simulink library "lib_controls"  (Simulink 7.9)
settings: Solver=ode45  SolverMode=SingleTasking  StartTime=0.0  StopTime=10.0  RelTol=1e-3
undefined symbols (not defined in the file): amb_tmp, cs_charge_deplete_bool, cs_charge_pwr, cs_charge_trq, cs_clt_tmp, cs_decel_fc_off, cs_decel_regen_threshold, cs_dl_assist_trq_threshold, cs_dl_regen_trq_threshold, cs_electric_decel_spd, cs_electric_launch_spd, cs_electric_launch_spd_hi, cs_electric_launch_spd_lo, cs_eng_min_spd, cs_eng_on_soc, cs_fc_init_state, cs_fc_max_pwr_frac, cs_fc_min_pwr_frac, cs_fc_on, cs_fc_pwr_opt, cs_fc_spd_opt, cs_fuzzy_fuel_mode, cs_hi_soc, cs_hi_trq_frac, cs_lo_soc, cs_lo_trq_frac, cs_max_gc_spd, cs_max_pwr, cs_max_pwr_fall_rate, cs_max_pwr_rise_rate, cs_mc_assist_max_frac, cs_mc_assist_min_frac, cs_mc_assist_slope, cs_mc_regen_max_frac, cs_mc_regen_min_frac, cs_mc_regen_slope, cs_mean_eff, cs_mean_eff_bool, cs_min_gc_spd, cs_min_off_time, cs_min_pwr, cs_min_trq_frac, cs_mph_avg_time, cs_off_trq_frac, cs_plot_output, cs_pwr, cs_regen_avg_time, cs_scale_factor, cs_shutoff, cs_soc_range, cs_spd, cs_target_soc, cs_trq_to_soc_factor, cvt_locus_pwr, cvt_locus_spd, cyc_mph, enable_sim_stop_distance, enable_sim_stop_max_spd, enable_sim_stop_speed, enable_sim_stop_time ... (+110)
libraries: lib_controls x124, simulink3 x18, lib_etc x1
(part 3 of 17)

== system lib_controls/electric assist control strategy bal <cs> ==
  "trq and spd req'd into clutch (N*m, rad/s)" : Inport
  Constant : Constant  Value=0
  MinMax : MinMax  Function=max  Inputs=2  SaturateOnIntegerOverflow=on  InputSameDT=on
  Mux : Mux  Inputs=2
  SOC corrected  trq req'd (N*m) : Subsystem
  Selector : Selector  InputPortWidth=2  IndexOptions=Index vector (dialog)  Indices=2  OutputSizes=1
  Switch : Switch  Threshold=eps  SaturateOnIntegerOverflow=on  InputSameDT=on
  help : Subsystem
      settings: OpenFcn=web(['file:\\\' which('Parallel.htm')])
      mask Display: image(imread('doc_man.jpg'))
  minimum trq (N*m) : Subsystem
  "trq and spd req'd from engine (N*m, rad/s)" : Outport
  wires:
  SOC corrected  trq req'd (N*m)/1(SOC corrected  trq req'd (N*m)) -> MinMax/1
  MinMax/1 -> Switch/1
  "trq and spd req'd into clutch (N*m, rad/s)"/1 -> SOC corrected  trq req'd (N*m)/1("trq and spd req'd into trq coupler (N*m, rad/s)"), Selector/1, minimum trq (N*m)/1("trq and spd req'd into trq coupler (N*m, rad/s)")
  minimum trq (N*m)/1(minimum trq (N*m)) -> MinMax/2
  [engine_on] -> Switch/2
  Selector/1 -> Mux/2
  Mux/1 -> "trq and spd req'd from engine (N*m, rad/s)"/1
  Switch/1 -> Mux/1
  Constant/1 -> Switch/3

== system lib_controls/electric assist control strategy  CVT <cs> ==
  "trq and spd req'd into clutch (N*m, rad/s)" : Inport
  Block NOTES1 : Subsystem
      mask Display: disp('Block\nNOTES')
  Constant : Constant  Value=0
  Demux : Demux  Outputs=2
  Demux1 : Demux  Outputs=2
  FC trq and spd : Subsystem
  MinMax : MinMax  Function=max  Inputs=2  SaturateOnIntegerOverflow=on  InputSameDT=on
  Mux : Mux  Inputs=2
  Switch : Switch  Threshold=eps  SaturateOnIntegerOverflow=on  InputSameDT=on
  To Workspace : ToWorkspace  VariableName=cl_trq_in_r  SampleTime=-1
  To Workspace1 : ToWorkspace  VariableName=cl_spd_in_r  SampleTime=-1
  To Workspace2 : ToWorkspace  VariableName=cs_trq_in_r  SampleTime=-1
  To Workspace3 : ToWorkspace  VariableName=cs_spd_in_r  SampleTime=-1
  help : Subsystem
      settings: OpenFcn=web(['file:\\\' which('Parallel.htm')])
      mask Display: image(imread('doc_man.jpg'))
  minimum trq (Nm) : Subsystem
  mod pwr req : Subsystem
  raw pwr req : Product  Inputs=1  SaturateOnIntegerOverflow=on  RndMeth=Zero  InputSameDT=on  OutDataTypeStr=Inherit: Same as first input
  "trq and spd req'd from engine (N*m, rad/s)" : Outport
  wires:
  Demux1/2 -> Mux/2, To Workspace1/1
  Demux/2 -> To Workspace3/1
  FC trq and spd/1("engine torque and speed (Nm), (rad/s)") -> Demux/1
  mod pwr req/1(Out1) -> FC trq and spd/1(power req'd by FC (W))
  Demux1/1 -> To Workspace/1
  "trq and spd req'd into clutch (N*m, rad/s)"/1 -> Demux1/1, minimum trq (Nm)/1("trq and spd req'd into trq coupler (N*m, rad/s)"), raw pwr req/1
  Switch/1 -> To Workspace2/1, Mux/1
  minimum trq (Nm)/1(minimum trq (N*m)) -> MinMax/1
  Demux/1 -> MinMax/2
  Mux/1 -> "trq and spd req'd from engine (N*m, rad/s)"/1
  Constant/1 -> Switch/3
  MinMax/1 -> Switch/1
  [mode] -> FC trq and spd/3(Mode)
  [engine_on] -> FC trq and spd/2(FC on), Switch/2
  raw pwr req/1 -> mod pwr req/1(In1)

== system lib_controls/fuel cell adaptive <cs> ==
  power req'd by bus (W) : Inport
  Delta SOC expected from regen : Subsystem
  Demux : Demux  Outputs=2
  Logical Operator : Logic
  Memory : Memory
  Minimize energy : S-Function  FunctionName=sfun_fuelcell_adapt  Parameters=cs_max_pwr_rise_rate,cs_max_pwr_fall_rate,fc_fuel_lhv,cs_shutoff,cs_min_pwr,cs_max_pwr,cs_mean_eff_bool,cs_mean_eff,cs_plot_output  EnableBusSupport=off
  Mux : Mux  Inputs=8
  SOC regulation factor : Subsystem
  engine pwr (W) : Outport
  tag scope: engine_on=global
  wires:
  power req'd by bus (W)/1 -> Mux/1, Delta SOC expected from regen/1(Power req'd by bus (W))
  Mux/1 -> Minimize energy/1
  [SOC] -> Mux/3, SOC regulation factor/1(In1), Delta SOC expected from regen/2(Soc)
  Minimize energy/1 -> Demux/1
  [key_on] -> Logical Operator/2
  Demux/2 -> Logical Operator/1
  Demux/1 -> engine pwr (W)/1
  Logical Operator/1 -> [engine_on]
  SOC regulation factor/1(Out1) -> Mux/4
  [ess_max_pwr] -> Mux/5
  [ess_max_chg_pwr] -> Mux/6
  [ess_tmp] -> Mux/7
  Memory/1 -> Mux/8
  [fc_pwr_out_a] -> Memory/1
  Delta SOC expected from regen/1(Delta SOC regen) -> Mux/2

== system lib_controls/fuel cell control strategy <cs> ==
  power req'd by bus (W) : Inport
  FC on : Subsystem
  "FC pwr command, modified by SOC" : Subsystem
  "FC pwr command, w/ limits enforced" : Subsystem
  Product : Product  SaturateOnIntegerOverflow=on  RndMeth=Zero  InputSameDT=on  OutDataTypeStr=Inherit: Same as first input
  Relational Operator : RelationalOperator  InputSameDT=on
  pwr req'd from FC to supply pwr req'd at bus (W) : Subsystem
  engine pwr (W) : Outport  InitialOutput=0
  tag scope: engine_on=global
  wires:
  power req'd by bus (W)/1 -> FC on/4(bus pwr req), "FC pwr command, modified by SOC"/3(pwr req'd at bus (W)), Relational Operator/1, pwr req'd from FC to supply pwr req'd at bus (W)/1(power req'd by bus (W))
  [ess_max_pwr] -> Relational Operator/2
  Product/1 -> engine pwr (W)/1
  pwr req'd from FC to supply pwr req'd at bus (W)/1(pwr req'd of FC (W)) -> "FC pwr command, modified by SOC"/2(raw pwr command (W))
  "FC pwr command, w/ limits enforced"/1(limited FC pwr command (W)) -> Product/2
  Relational Operator/1 -> FC on/1(ess max pwr would be insufficient), "FC pwr command, w/ limits enforced"/1(ess max pwr would be insufficient)
  [SOC] -> "FC pwr command, modified by SOC"/1(SOC), FC on/2(SOC), "FC pwr command, w/ limits enforced"/2(SOC)
  "FC pwr command, modified by SOC"/1(pwr command modifed for SOC (W)) -> "FC pwr command, w/ limits enforced"/3(FC pwr command), FC on/3(FC pwr command)
  FC on/1(FC on) -> [engine_on], Product/1

== system lib_controls/fuel cell <cs> config ==
  power req'd by bus (W) : Inport
  fuel cell adaptive <cs> : lib_controls/fuel cell adaptive <cs>
  engine pwr (W) : Outport
  wires:
  power req'd by bus (W)/1 -> fuel cell adaptive <cs>/1
  fuel cell adaptive <cs>/1 -> engine pwr (W)/1

== system lib_controls/par <cs> config ==
  "trq and spd req'd into clutch (N*m, rad/s)" : Inport
  electric assist control strategy <cs> : lib_controls/electric assist control strategy <cs>
  "trq and spd req'd from engine (N*m, rad/s)" : Outport
  wires:
  "trq and spd req'd into clutch (N*m, rad/s)"/1 -> electric assist control strategy <cs>/1
  electric assist control strategy <cs>/1 -> "trq and spd req'd from engine (N*m, rad/s)"/1

== system lib_controls/par <vc> config ==
  <vc> par : lib_controls/<vc> par
  clutch state : Outport
  wires:
  <vc> par/1 -> clutch state/1

== system lib_controls/series hybrid control stategy  <cs> ==
  power req'd by bus (W) : Inport
  FC on : Subsystem
  "FC pwr command, modified by SOC" : Subsystem
  "FC pwr command, w/ limits enforced" : Subsystem
  FC trq and spd : Subsystem
  Relational Operator : RelationalOperator  InputSameDT=on
  Selector : Selector  InputPortWidth=2  IndexOptions=Index vector (dialog)  Indices=2  OutputSizes=1
  power follower : Subsystem
      settings: OpenFcn=web(['file:\\\' which('Series.htm')]);
      mask Display: image(imread('doc_man.jpg'))
  pwr req'd from FC to supply pwr req'd at bus (W) : Subsystem
  thermostat : Subsystem
      settings: OpenFcn=web(['file:\\\' which('Series-therm.htm')]);
      mask Display: image(imread('doc_man.jpg'))
  "engine torque and speed (Nm), (rad/s)" : Outport  InitialOutput=0
  tag scope: engine_on=global, spd_command=global
  wires:
  Selector/1 -> [spd_command]
  FC trq and spd/1("engine torque and speed (Nm), (rad/s)") -> Selector/1, "engine torque and speed (Nm), (rad/s)"/1
  "FC pwr command, w/ limits enforced"/1(limited FC pwr command (W)) -> FC trq and spd/2(power req'd by FC (W))
  FC on/1(FC on) -> [engine_on], FC trq and spd/1(FC on)
  power req'd by bus (W)/1 -> FC on/4(bus pwr req), "FC pwr command, modified by SOC"/3(pwr req'd at bus (W)), Relational Operator/1, pwr req'd from FC to supply pwr req'd at bus (W)/1(power req'd by bus (W))
  [ess_max_pwr] -> Relational Operator/2
  Relational Operator/1 -> FC on/1(ess max pwr would be insufficient), "FC pwr command, w/ limits enforced"/1(ess max pwr would be insufficient)
  pwr req'd from FC to supply pwr req'd at bus (W)/1(pwr req'd of FC (W)) -> "FC pwr command, modified by SOC"/2(raw pwr command (W))
  "FC pwr command, modified by SOC"/1(pwr command modifed for SOC (W)) -> "FC pwr command, w/ limits enforced"/3(FC pwr command), FC on/3(FC pwr command)
  [SOC] -> FC on/2(SOC), "FC pwr command, w/ limits enforced"/2(SOC), "FC pwr command, modified by SOC"/1(SOC)

== system lib_controls/user contributed engine on (balanced parallel hybrid) ==
  trq req'd out of clutch (N*m) : Inport
  spd req'd out of clutch (N*m)1 : Inport  Port=2
  fc_spd_out_r : Inport  Port=3
  v_ave_req : Inport  Port=4
  clutch state : Inport  Port=5
  (--)2 : Constant  Value=fc_on
  (--)3 : Constant
  (--)4 : Constant  Value=cs_lo_soc
  Block NOTES : Subsystem
      mask Display: disp('Block\nNOTES')
  Constant1 : Constant  Value=vc_eng_warmup_time
  Constant2 : Constant  Value=engine_shutdown_delay
  Constant3 : Constant  Value=vc_launch_spd
  Constant4 : Constant
  Constant{5..7,9} (4 alike) : Constant  Value=0
  Constant8 : Constant
  Hit  Crossing1 : HitCross  HitCrossingDirection=rising
  Logical Operator10 : Logic  Inputs=3
  Logical Operator12 : Logic  Inputs=3
  Logical Operator2 : Logic
  Rate Limiter1 : RateLimiter  RisingSlewLimit=inf  FallingSlewLimit=-1/1
  Relational Operator1 : RelationalOperator  Operator=>  InputSameDT=on
  Saturation : Saturate  UpperLimit=max(fc_map_spd)*fc_spd_scale  LowerLimit=vc_idle_spd*vc_idle_bool
  Switch{,1..4} (5 alike) : Switch  Threshold=eps  SaturateOnIntegerOverflow=on  InputSameDT=on
  Terminator : Terminator
  Terminator1 : Terminator
  clutch disengaged : RelationalOperator  Operator===  InputSameDT=on
  clutch disengaged1 : RelationalOperator  Operator===  InputSameDT=on
  key_on : lib_controls/<vc> ISG bal shift by time CD3xx/engine on (balanced parallel hybrid)/key_on  MaskParam1=vc_key_on(:,1)  MaskParam2=vc_key_on(:,2)
  moving next time : RelationalOperator  Operator=>  InputSameDT=on
  moving next time1 : RelationalOperator  InputSameDT=on
  not moving : RelationalOperator  Operator===  InputSameDT=on
  repeated cycle time : lib_controls/<vc> ISG bal shift by time CD3xx/engine on (balanced parallel hybrid)/repeated cycle time  t=cyc_mph(:,1)  y=cyc_mph(:,1)
  repeated cycle:  speed required at end of NEXT step : lib_controls/<vc> ISG bal shift by time CD3xx/engine on (balanced parallel hybrid)/repeated cycle:  speed required at end of NEXT step  t=cyc_mph(:,1)  y=cyc_mph(:,2)
  engine on : Outport
  spd command  (rad/s) : Outport  Port=2
  key on : Outport  Port=3
  wires:
  trq req'd out of clutch (N*m)/1 -> Terminator/1
  spd req'd out of clutch (N*m)1/1 -> Terminator1/1
  Logical Operator2/1 -> Switch3/2
  Relational Operator1/1 -> Logical Operator2/2
  Switch3/1 -> Logical Operator12/3
  moving next time1/1 -> Logical Operator2/1
  (--)3/1 -> Switch3/3
  Constant1/1 -> Relational Operator1/2
  repeated cycle time/1 -> Relational Operator1/1
  [SOC] -> moving next time1/1
  key_on/1 -> Logical Operator12/2, key on/1  "ignition key is on"
  (--)2/1 -> Logical Operator12/1
  Constant3/1 -> Switch/1
  Switch/1 -> Saturation/1
  Logical Operator10/1 -> Switch/2
  fc_spd_out_r/1 -> Switch/3
  Saturation/1 -> Switch1/1
  clutch state/1 -> clutch disengaged/1
  Switch1/1 -> spd command  (rad/s)/1
  Constant7/1 -> Switch1/3
  Constant4/1 -> clutch disengaged/2
  v_ave_req/1 -> not moving/1
  Constant5/1 -> not moving/2
  repeated cycle:  speed required at end of NEXT step/1 -> moving next time/1, Switch2/2, clutch disengaged1/1
  Constant6/1 -> moving next time/2
  clutch disengaged/1 -> Logical Operator10/1
  not moving/1 -> Logical Operator10/2
  moving next time/1 -> Logical Operator10/3, Switch4/2
  (--)4/1 -> moving next time1/2
  Logical Operator12/1 -> Switch4/3
  Constant8/1 -> Switch4/1
  Switch4/1 -> engine on/1, Switch1/2
  Switch2/1 -> Switch3/1
  Constant2/1 -> Switch2/1
  Constant9/1 -> clutch disengaged1/2
  clutch disengaged1/1 -> Hit  Crossing1/1
  Hit  Crossing1/1 -> Rate Limiter1/1
  Rate Limiter1/1 -> Switch2/3

== system lib_controls/<vc> conv/clutch control ==
  shifting : Inport
  gb_trq_in_r : Inport  Port=2
  gb_spd_in_r : Inport  Port=3
  Block NOTES : Subsystem
      mask Display: disp('Block\nNOTES')
  Constant : Constant  Value=1e-3
  Constant1 : Constant  Value=vc_clutch_bool
  Constant2 : Constant  Value=vc_idle_spd
  Constant3 : Constant  Value=1e-3
  Constant4 : Constant  Value=vc_launch_spd
  Constant5 : Constant  Value=2.5
  Fcn: 1 if clutch disengaged 2 if clutch slipping 3 if clutch engaged : Fcn  Expr=u[1]+2*u[2]*(1-u[1])*(1-u[3])+3*u[3]*(1-u[1])
  Logical Operator : Logic
  Logical Operator1 : Logic  Operator=OR
  Memory : Memory  X0=1+(2*(cyc_mph(1,2)>0))
  Mux : Mux  Inputs=3
  Relational Operator : RelationalOperator  Operator=<=  InputSameDT=on
  Relational Operator1 : RelationalOperator  Operator=<  InputSameDT=on
  Relational Operator2 : RelationalOperator  Operator=>  InputSameDT=on
  Relational Operator3 : RelationalOperator  Operator=<  InputSameDT=on
  clutch disengaged : Logic  Operator=OR
  clutch engaged : Logic  Operator=NOR
  clutch slipping : Logic  Inputs=3
  clutch was NOT fully engaged during last time step : RelationalOperator  Operator=<  InputSameDT=on
  gearbox speed estimator : Subsystem
  clutch state : Outport
  wires:
  gearbox speed estimator/1(Out1) -> Relational Operator3/1, Relational Operator1/1
  gb_spd_in_r/1 -> gearbox speed estimator/1(gb_spd_in_r if no gear change)
  shifting/1 -> clutch disengaged/1
  Logical Operator/1 -> clutch disengaged/2
  gb_trq_in_r/1 -> Relational Operator2/1, Relational Operator/1
  Logical Operator1/1 -> Logical Operator/2
  Relational Operator/1 -> Logical Operator/1
  Constant/1 -> Relational Operator/2
  Constant1/1 -> Logical Operator1/1
  clutch was NOT fully engaged during last time step/1 -> clutch slipping/3
  Constant5/1 -> clutch was NOT fully engaged during last time step/2
  Memory/1 -> clutch was NOT fully engaged during last time step/1
  Relational Operator3/1 -> clutch slipping/2
  Constant4/1 -> Relational Operator3/2
  clutch slipping/1 -> Mux/2, clutch engaged/2
  Relational Operator2/1 -> clutch slipping/1
  Constant3/1 -> Relational Operator2/2
  Fcn: 1 if clutch disengaged 2 if clutch slipping 3 if clutch engaged/1 -> Memory/1, clutch state/1
  clutch disengaged/1 -> Mux/1, clutch engaged/1
  clutch engaged/1 -> Mux/3
  Mux/1 -> Fcn: 1 if clutch disengaged 2 if clutch slipping 3 if clutch engaged/1
  Constant2/1 -> Relational Operator1/2
  Relational Operator1/1 -> Logical Operator1/2

== system lib_controls/<vc> conv/config traction control ==
  time-average vehicle speed  req'd (m/s) : Inport
  vehicle speed at beginning of time  step (m/s) : Inport  Port=2
  total tractive force req'd (N) : Inport  Port=3
  traction control 2 axle : lib_controls/SubSystem/traction control 2 axle
  req'd force (N) : Outport
  req'd speed (m/s) : Outport  Port=2
  weight on front axle (N) : Outport  Port=3
  weight on rear axle (N) : Outport  Port=4
  front/total  traction ratio : Outport  Port=5
  wires:
  time-average vehicle speed  req'd (m/s)/1 -> traction control 2 axle/1
  vehicle speed at beginning of time  step (m/s)/1 -> traction control 2 axle/2
  total tractive force req'd (N)/1 -> traction control 2 axle/3
  traction control 2 axle/1 -> req'd force (N)/1
  traction control 2 axle/2 -> req'd speed (m/s)/1
  traction control 2 axle/3 -> weight on front axle (N)/1
  traction control 2 axle/4 -> weight on rear axle (N)/1
  traction control 2 axle/5 -> front/total  traction ratio/1

== system lib_controls/<vc> conv/engine control ==
  clutch state : Inport
  shifting : Inport  Port=2
  fc_spd_out_r : Inport  Port=3
  v_ave_req : Inport  Port=4
  Block NOTES : Subsystem
      mask Display: disp('Block\nNOTES')
  Constant : Constant  Value=1.1
  Constant1 : Constant  Value=vc_idle_bool
  Constant2 : Constant  Value=vc_launch_spd
  Constant3 : Constant
  Constant4 : Constant  Value=0
  Constant5 : Constant  Value=0
  Constant6 : Constant  Value=0
  Logical Operator1 : Logic
  Logical Operator2 : Logic  Operator=OR
  Logical Operator3 : Logic  Operator=OR
  Logical Operator7 : Logic
  Logical Operator8 : Logic  Inputs=3
  Memory : Memory
  Saturation : Saturate  UpperLimit=max(fc_map_spd)*fc_spd_scale  LowerLimit=vc_idle_spd*vc_idle_bool
  Switch : Switch  Threshold=eps  SaturateOnIntegerOverflow=on  InputSameDT=on
  Switch1 : Switch  Threshold=eps  SaturateOnIntegerOverflow=on  InputSameDT=on
  clutch disengaged : RelationalOperator  Operator===  InputSameDT=on
  clutch slipping or engaged : RelationalOperator  Operator=>  InputSameDT=on
  key_on : Subsystem  mask(Repeating table){t=vc_key_on(:,1), y=vc_key_on(:,2)}
      mask prompts: t "Time values:"; y "Output values:"
      mask help:
      | Repeating table.
      | Enter values of time and output for first cycle.
      mask init:
      | period = max(t);
      mask Help: Repeats cycle given in table. Time values should be monotonically increasing.
  moving next time : RelationalOperator  Operator=>  InputSameDT=on
  not moving : RelationalOperator  Operator===  InputSameDT=on
  repeated cycle:  speed required at end of NEXT step : Subsystem  mask(Forward looking repeating table){t=cyc_mph(:,1), y=cyc_mph(:,2)}
      mask prompts: t "Time values:"; y "Output values:"
      mask help:
      | Forward looking repeating table.
      | Enter values of time and output for first cycle.
      mask init:
      | period = max(t);
      mask Help: Repeats cycle given in table with a one time step forward offset. Time values should be monotonically increasing.
  engine on : Outport
  spd command  (rad/s) : Outport  Port=2
  key on : Outport  Port=3
  wires:
  key_on/1(out_1) -> key on/1, Logical Operator1/1
  Constant6/1 -> Switch1/3
  Switch1/1 -> spd command  (rad/s)/1
  Saturation/1 -> Switch1/1
  Logical Operator3/1 -> Switch1/2, Memory/1, engine on/1
  Switch/1 -> Saturation/1
  Constant2/1 -> Switch/1
  fc_spd_out_r/1 -> Switch/3
  Logical Operator8/1 -> Switch/2
  Constant4/1 -> not moving/2
  Constant3/1 -> clutch disengaged/2
  v_ave_req/1 -> not moving/1
  repeated cycle:  speed required at end of NEXT step/1(out_1) -> moving next time/1
  Constant5/1 -> moving next time/2
  Logical Operator7/1 -> Logical Operator3/2
  Memory/1 -> Logical Operator7/2
  shifting/1 -> Logical Operator7/1
  Logical Operator2/1 -> Logical Operator1/2
  Logical Operator1/1 -> Logical Operator3/1
  clutch slipping or engaged/1 -> Logical Operator2/1
  Constant/1 -> clutch slipping or engaged/2
  Constant1/1 -> Logical Operator2/2
  clutch state/1 -> clutch slipping or engaged/1, clutch disengaged/1
  moving next time/1 -> Logical Operator8/3
  not moving/1 -> Logical Operator8/2
  clutch disengaged/1 -> Logical Operator8/1

== system lib_controls/<vc> conv/gearbox  control ==
  note: default gear number
      | calculation
  note: default shifting
      | calculation
  note: default gear ratio
      | calculation
  note: gear ratio and shifting pre-muxed
  note: output changes depending
      | upon whether speed
      | dependent shifting is used
  note: local GOTO blocks:
  note: local GOTO blocks
  gb_trq_out_r : Inport
  gb_spd_out_r : Inport  Port=2
  prev. Pout/Pin : Inport  Port=3
  tires are at traction limit : Inport  Port=4
  Block NOTES : Subsystem
      mask Display: disp('Block\nNOTES')
  Constant : Constant
  Constant14 : Constant  Value=tx_speed_dep
  Constant15 : Constant  Value=tx_speed_dep
  Demux : Demux  Outputs=2
  Fcn : Fcn  Expr=1/u
  Fcn1 : Fcn  Expr=1/u
  Gain1 : Gain  Gain=-1  SaturateOnIntegerOverflow=on  OutDataTypeStr=Inherit: Same as input  ParamDataTypeStr=Inherit: Same as input
  Mux : Mux  Inputs=2
  Product2 : Product  Inputs=*/  SaturateOnIntegerOverflow=on  RndMeth=Zero  InputSameDT=on  OutDataTypeStr=Inherit: Same as first input
  Product3 : Product  SaturateOnIntegerOverflow=on  RndMeth=Zero  InputSameDT=on  OutDataTypeStr=Inherit: Same as first input
  Rate Limiter : RateLimiter  RisingSlewLimit=1/(gb_shift_delay+eps)  FallingSlewLimit=-1/(gb_shift_delay+eps)
  Saturation : Saturate  UpperLimit=1  LowerLimit=0.2
  Saturation1 : Saturate  UpperLimit=gb_gears_num  LowerLimit=1
  Speed Dependent Shifting : lib_controls/SubSystem/Speed Dependent Shifting
      settings: RTWFcnNameOpts=Auto  RTWFileNameOpts=Auto
  Switch : Switch  Threshold=eps  SaturateOnIntegerOverflow=on  InputSameDT=on
  Switch1 : Switch  Threshold=0.5  SaturateOnIntegerOverflow=on  InputSameDT=on
  Switch2 : Switch  Threshold=0.5  SaturateOnIntegerOverflow=on  InputSameDT=on
  allow downshift? : Subsystem
  current gear number : Sum  SaturateOnIntegerOverflow=on  InputSameDT=on  OutDataTypeStr=Inherit: Same as first input
  delta gear number : Switch  Threshold=eps  SaturateOnIntegerOverflow=on  InputSameDT=on
  downshift  command : Subsystem
  engine torque capability : Lookup  InputValues=fc_map_spd*fc_spd_scale  Table=fc_max_trq*fc_trq_scale+eps  SaturateOnIntegerOverflow=on
  est eng trq : Sum  SaturateOnIntegerOverflow=on  InputSameDT=on  OutDataTypeStr=Inherit: Same as first input
  gb_spd_in_r : Product  SaturateOnIntegerOverflow=on  RndMeth=Zero  InputSameDT=on  OutDataTypeStr=Inherit: Same as first input
  gear ratio : Lookup  InputValues=[1:length(gb_ratio)]  Table=gb_ratio  SaturateOnIntegerOverflow=on
  gear ratio1 : Lookup  InputValues=[1:length(gb_ratio)]  Table=gb_ratio  SaturateOnIntegerOverflow=on
  gearbox speed estimator : Subsystem
  load=T/ (maxT at spd) : Saturate  UpperLimit=1  LowerLimit=0
  prev gear number : Memory  X0=gb_num_init
  prev gear ratio : Memory  X0=gb_ratio(gb_num_init)
  shifting1 : Subsystem
  upshift  command : Subsystem
  ~gb_trq_in_r : Product  Inputs=3  SaturateOnIntegerOverflow=on  RndMeth=Zero  InputSameDT=on  OutDataTypeStr=Inherit: Same as first input
  "gear ratio, out" : Outport  InitialOutput=0
  "shifting, out" : Outport  Port=2  InitialOutput=0
  "gear number, out" : Outport  Port=3  InitialOutput=0
  wires:
  delta gear number/1 -> current gear number/2
  Switch/1 -> downshift  command/2(engine load), upshift  command/2(engine load)
  load=T/ (maxT at spd)/1 -> Switch/3
  est eng trq/1 -> Product2/1
  ~gb_trq_in_r/1 -> est eng trq/1
  gearbox speed estimator/1(Out1) -> upshift  command/3(engine speed), downshift  command/3(engine speed), engine torque capability/1
  allow downshift?/1(allow shift) -> Product3/1
  Product3/1 -> delta gear number/3
  Gain1/1 -> Product3/2
  prev gear ratio/1 -> Fcn1/1, gb_spd_in_r/2
  gear ratio/1 -> prev gear ratio/1
  gb_spd_in_r/1 -> gearbox speed estimator/1(gb_spd_in_r if no gear change)
  gb_spd_out_r/1 -> gb_spd_in_r/1
  Rate Limiter/1 -> gear ratio/1
  tires are at traction limit/1 -> Switch/2
  Constant/1 -> Switch/1
  Product2/1 -> load=T/ (maxT at spd)/1
  prev gear number/1 -> current gear number/1, downshift  command/1(prev gear number), upshift  command/1(prev gear number), allow downshift?/1(prev gearnum)
  Saturation1/1 -> shifting1/1(gear number), Rate Limiter/1, [def_gear_num], gear ratio1/1, prev gear number/1
  Fcn/1 -> ~gb_trq_in_r/2
  engine torque capability/1 -> Product2/2
  Fcn1/1 -> ~gb_trq_in_r/3
  downshift  command/1(command) -> Gain1/1
  upshift  command/1(command) -> delta gear number/2, delta gear number/1
  gb_trq_out_r/1 -> ~gb_trq_in_r/1
  prev. Pout/Pin/1 -> Saturation/1
  Saturation/1 -> Fcn/1
  current gear number/1 -> Saturation1/1
  gear ratio1/1 -> [def_gear_ratio]
  shifting1/1(out_1) -> [def_shifting]
  Constant15/1 -> Switch2/2
  [spd_dep_muxed] -> Switch2/1
  Mux/1 -> Switch2/3
  [def_gear_ratio] -> Mux/1
  [def_shifting] -> Mux/2
  [v_req_limited] -> Speed Dependent Shifting/1
  Speed Dependent Shifting/1 -> [spd_dep_muxed]
  Speed Dependent Shifting/2 -> [spd_dep_gear_num]
  Switch2/1 -> Demux/1
  Demux/1 -> "gear ratio, out"/1
  Demux/2 -> "shifting, out"/1
  Switch1/1 -> "gear number, out"/1
  Constant14/1 -> Switch1/2
  [spd_dep_gear_num] -> Switch1/1
  [def_gear_num] -> Switch1/3
  [acc_mech_trq_est] -> est eng trq/2

== system lib_controls/<vc> conv Saber custom/clutch control ==
  shifting : Inport
  gb_trq_in_r : Inport  Port=2
  gb_spd_in_r : Inport  Port=3
  Block NOTES : Subsystem
      mask Display: disp('Block\nNOTES')
  Constant : Constant  Value=1e-3
  Constant1 : Constant  Value=vc_clutch_bool
  Constant2 : Constant  Value=vc_idle_spd
  Constant3 : Constant  Value=1e-3
  Constant4 : Constant  Value=vc_launch_spd
  Constant5 : Constant  Value=2.5
  Fcn: 1 if clutch disengaged 2 if clutch slipping 3 if clutch engaged : Fcn  Expr=u[1]+2*u[2]*(1-u[1])*(1-u[3])+3*u[3]*(1-u[1])
  Logical Operator : Logic
  Logical Operator1 : Logic  Operator=OR
  Memory : Memory  X0=1+(2*(cyc_mph(1,2)>0))
  Mux : Mux  Inputs=3
  Relational Operator : RelationalOperator  Operator=<=  InputSameDT=on
  Relational Operator1 : RelationalOperator  Operator=<  InputSameDT=on
  Relational Operator2 : RelationalOperator  Operator=>  InputSameDT=on
  Relational Operator3 : RelationalOperator  Operator=<  InputSameDT=on
  clutch disengaged : Logic  Operator=OR
  clutch engaged : Logic  Operator=NOR
  clutch slipping : Logic  Inputs=3
  clutch was NOT fully engaged during last time step : RelationalOperator  Operator=<  InputSameDT=on
  gearbox speed estimator : Subsystem
  clutch state : Outport
  wires:
  Relational Operator1/1 -> Logical Operator1/2
  Constant2/1 -> Relational Operator1/2
  Mux/1 -> Fcn: 1 if clutch disengaged 2 if clutch slipping 3 if clutch engaged/1
  clutch engaged/1 -> Mux/3
  clutch disengaged/1 -> clutch engaged/1, Mux/1
  Fcn: 1 if clutch disengaged 2 if clutch slipping 3 if clutch engaged/1 -> clutch state/1, Memory/1
  Constant3/1 -> Relational Operator2/2
  Relational Operator2/1 -> clutch slipping/1
  clutch slipping/1 -> clutch engaged/2, Mux/2
  Constant4/1 -> Relational Operator3/2
  Relational Operator3/1 -> clutch slipping/2
  Memory/1 -> clutch was NOT fully engaged during last time step/1
  Constant5/1 -> clutch was NOT fully engaged during last time step/2
  clutch was NOT fully engaged during last time step/1 -> clutch slipping/3
  Constant1/1 -> Logical Operator1/1
  Constant/1 -> Relational Operator/2
  Relational Operator/1 -> Logical Operator/1
  Logical Operator1/1 -> Logical Operator/2
  gb_trq_in_r/1 -> Relational Operator/1, Relational Operator2/1
  Logical Operator/1 -> clutch disengaged/2
  shifting/1 -> clutch disengaged/1
  gb_spd_in_r/1 -> gearbox speed estimator/1(gb_spd_in_r if no gear change)
  gearbox speed estimator/1(Out1) -> Relational Operator1/1, Relational Operator3/1

== system lib_controls/<vc> conv Saber custom/config traction control ==
  time-average vehicle speed  req'd (m/s) : Inport
  vehicle speed at beginning of time  step (m/s) : Inport  Port=2
  total tractive force req'd (N) : Inport  Port=3
  traction control 2 axle : lib_controls/SubSystem/traction control 2 axle
      settings: RTWFcnNameOpts=Auto  RTWFileNameOpts=Auto
  req'd force (N) : Outport
  req'd speed (m/s) : Outport  Port=2
  weight on front axle (N) : Outport  Port=3
  weight on rear axle (N) : Outport  Port=4
  front/total  traction ratio : Outport  Port=5
  wires:
  time-average vehicle speed  req'd (m/s)/1 -> traction control 2 axle/1
  vehicle speed at beginning of time  step (m/s)/1 -> traction control 2 axle/2
  total tractive force req'd (N)/1 -> traction control 2 axle/3
  traction control 2 axle/1 -> req'd force (N)/1
  traction control 2 axle/2 -> req'd speed (m/s)/1
  traction control 2 axle/3 -> weight on front axle (N)/1
  traction control 2 axle/4 -> weight on rear axle (N)/1
  traction control 2 axle/5 -> front/total  traction ratio/1

== system lib_controls/<vc> conv Saber custom/engine control ==
  clutch state : Inport
  shifting : Inport  Port=2
  fc_spd_out_r : Inport  Port=3
  v_ave_req : Inport  Port=4
  Block NOTES : Subsystem
      mask Display: disp('Block\nNOTES')
  Constant : Constant  Value=1.1
  Constant1 : Constant  Value=vc_idle_bool
  Constant2 : Constant  Value=vc_launch_spd
  Constant3 : Constant
  Constant4 : Constant  Value=0
  Constant5 : Constant  Value=0
  Constant6 : Constant  Value=0
  Logical Operator1 : Logic
  Logical Operator2 : Logic  Operator=OR
  Logical Operator3 : Logic  Operator=OR
  Logical Operator7 : Logic
  Logical Operator8 : Logic  Inputs=3
  Memory : Memory
  Saturation : Saturate  UpperLimit=max(fc_map_spd)*fc_spd_scale  LowerLimit=vc_idle_spd*vc_idle_bool
  Switch : Switch  Threshold=eps  SaturateOnIntegerOverflow=on  InputSameDT=on
  Switch1 : Switch  Threshold=eps  SaturateOnIntegerOverflow=on  InputSameDT=on
  clutch disengaged : RelationalOperator  Operator===  InputSameDT=on
  clutch slipping or engaged : RelationalOperator  Operator=>  InputSameDT=on
  key_on : Subsystem  mask(Repeating table){@1=vc_key_on(:,1), @2=vc_key_on(:,2)}
      mask prompts: @1 "Time values:"; @2 "Output values:"
      mask help:
      | Repeating table.
      | Enter values of time and output for first cycle.
      mask init:
      | period = max(@1); t = @1; y = @2;
      mask Help: Repeats cycle given in table. Time values should be monotonically increasing.
  moving next time : RelationalOperator  Operator=>  InputSameDT=on
  not moving : RelationalOperator  Operator===  InputSameDT=on
  repeated cycle:  speed required at end of NEXT step : Subsystem  mask(Forward looking repeating table){t=cyc_mph(:,1), y=cyc_mph(:,2)}
      mask prompts: t "Time values:"; y "Output values:"
      mask help:
      | Forward looking repeating table.
      | Enter values of time and output for first cycle.
      mask init:
      | period = max(t);
      mask Help: Repeats cycle given in table with a one time step forward offset. Time values should be monotonically increasing.
  engine on : Outport
  spd command  (rad/s) : Outport  Port=2
  key on : Outport  Port=3
  wires:
  clutch disengaged/1 -> Logical Operator8/1
  not moving/1 -> Logical Operator8/2
  moving next time/1 -> Logical Operator8/3
  clutch state/1 -> clutch disengaged/1, clutch slipping or engaged/1
  Constant1/1 -> Logical Operator2/2
  Constant/1 -> clutch slipping or engaged/2
  clutch slipping or engaged/1 -> Logical Operator2/1
  Logical Operator1/1 -> Logical Operator3/1
  Logical Operator2/1 -> Logical Operator1/2
  shifting/1 -> Logical Operator7/1
  Memory/1 -> Logical Operator7/2
  Logical Operator7/1 -> Logical Operator3/2
  Constant5/1 -> moving next time/2
  repeated cycle:  speed required at end of NEXT step/1(out_1) -> moving next time/1
  v_ave_req/1 -> not moving/1
  Constant3/1 -> clutch disengaged/2
  Constant4/1 -> not moving/2
  Logical Operator8/1 -> Switch/2
  fc_spd_out_r/1 -> Switch/3
  Constant2/1 -> Switch/1
  Switch/1 -> Saturation/1
  Logical Operator3/1 -> engine on/1, Memory/1, Switch1/2
  Saturation/1 -> Switch1/1
  Switch1/1 -> spd command  (rad/s)/1
  Constant6/1 -> Switch1/3
  key_on/1(out_1) -> Logical Operator1/1, key on/1

== system lib_controls/<vc> conv Saber custom/gearbox  control ==
  note: gear ratio and shifting pre-muxed
  note: output changes depending
      | upon whether speed
      | dependent shifting is used
  note: default gear number
      | calculation
  note: default gear ratio
      | calculation
  note: local GOTO blocks:
  gb_trq_out_r : Inport
  gb_spd_out_r : Inport  Port=2
  prev. Pout/Pin : Inport  Port=3
  tires are at traction limit : Inport  Port=4
  Block NOTES : Subsystem
      mask Display: disp('Block\nNOTES')
  Constant : Constant
  Constant14 : Constant  Value=tx_speed_dep
  Constant15 : Constant  Value=tx_speed_dep
  Demux : Demux  Outputs=2
  Fcn : Fcn  Expr=1/u
  Fcn1 : Fcn  Expr=1/u
  Gain1 : Gain  Gain=-1  SaturateOnIntegerOverflow=on  OutDataTypeStr=Inherit: Same as input  ParamDataTypeStr=Inherit: Same as input
  Mux : Mux  Inputs=2
  Product2 : Product  Inputs=*/  SaturateOnIntegerOverflow=on  RndMeth=Zero  InputSameDT=on  OutDataTypeStr=Inherit: Same as first input
  Product3 : Product  SaturateOnIntegerOverflow=on  RndMeth=Zero  InputSameDT=on  OutDataTypeStr=Inherit: Same as first input
  Rate Limiter : RateLimiter  RisingSlewLimit=1/(gb_shift_delay+eps)  FallingSlewLimit=-1/(gb_shift_delay+eps)
  Saturation : Saturate  UpperLimit=1  LowerLimit=0.2
  Saturation1 : Saturate  UpperLimit=gb_gears_num  LowerLimit=1
  Speed Dependent Shifting : lib_controls/SubSystem/Speed Dependent Shifting
      settings: RTWFcnNameOpts=Auto  RTWFileNameOpts=Auto
  Switch : Switch  Threshold=eps  SaturateOnIntegerOverflow=on  InputSameDT=on
  Switch2 : Switch  Threshold=0.5  SaturateOnIntegerOverflow=on  InputSameDT=on
  Switch3 : Switch  Threshold=0.5  SaturateOnIntegerOverflow=on  InputSameDT=on
  accessories (Nm) : Subsystem
  allow downshift? : Subsystem
  current gear number : Sum  SaturateOnIntegerOverflow=on  InputSameDT=on  OutDataTypeStr=Inherit: Same as first input
  delta gear number : Switch  Threshold=eps  SaturateOnIntegerOverflow=on  InputSameDT=on
  downshift  command : Subsystem
  engine torque capability : Lookup  InputValues=fc_map_spd*fc_spd_scale  Table=fc_max_trq*fc_trq_scale+eps  SaturateOnIntegerOverflow=on
  est eng trq : Sum  SaturateOnIntegerOverflow=on  InputSameDT=on  OutDataTypeStr=Inherit: Same as first input
  gb_spd_in_r : Product  SaturateOnIntegerOverflow=on  RndMeth=Zero  InputSameDT=on  OutDataTypeStr=Inherit: Same as first input
  gear ratio : Lookup  InputValues=[1:length(gb_ratio)]  Table=gb_ratio  SaturateOnIntegerOverflow=on
  gear ratio1 : Lookup  InputValues=[1:length(gb_ratio)]  Table=gb_ratio  SaturateOnIntegerOverflow=on
  gearbox speed estimator : Subsystem
  load=T/ (maxT at spd) : Saturate  UpperLimit=1  LowerLimit=0
  prev gear number : Memory  X0=gb_num_init
  prev gear ratio : Memory  X0=gb_ratio(gb_num_init)
  shifting1 : Subsystem
  upshift  command : Subsystem
  ~gb_trq_in_r : Product  Inputs=3  SaturateOnIntegerOverflow=on  RndMeth=Zero  InputSameDT=on  OutDataTypeStr=Inherit: Same as first input
  "gear ratio, out" : Outport  InitialOutput=0
  "shifting, out" : Outport  Port=2  InitialOutput=0
  "gear number, out" : Outport  Port=3  InitialOutput=0
  wires:
  current gear number/1 -> Saturation1/1
  Saturation/1 -> Fcn/1
  prev. Pout/Pin/1 -> Saturation/1
  gb_trq_out_r/1 -> ~gb_trq_in_r/1
  upshift  command/1(command) -> delta gear number/1, delta gear number/2
  downshift  command/1(command) -> Gain1/1
  Fcn1/1 -> ~gb_trq_in_r/3
  engine torque capability/1 -> Product2/2
  Fcn/1 -> ~gb_trq_in_r/2
  Saturation1/1 -> prev gear number/1, gear ratio1/1, [def_gear_num], Rate Limiter/1, shifting1/1(gear number)
  prev gear number/1 -> allow downshift?/1(prev gearnum), upshift  command/1(prev gear number), downshift  command/1(prev gear number), current gear number/1
  Product2/1 -> load=T/ (maxT at spd)/1
  Constant/1 -> Switch/1
  tires are at traction limit/1 -> Switch/2
  Rate Limiter/1 -> gear ratio/1
  gb_spd_out_r/1 -> gb_spd_in_r/1
  gb_spd_in_r/1 -> gearbox speed estimator/1(gb_spd_in_r if no gear change)
  gear ratio/1 -> prev gear ratio/1
  prev gear ratio/1 -> gb_spd_in_r/2, Fcn1/1
  Gain1/1 -> Product3/2
  Product3/1 -> delta gear number/3
  allow downshift?/1(allow shift) -> Product3/1
  ~gb_trq_in_r/1 -> est eng trq/1
  accessories (Nm)/1(T_acc) -> est eng trq/2
  est eng trq/1 -> Product2/1
  load=T/ (maxT at spd)/1 -> Switch/3
  Switch/1 -> upshift  command/2(engine load), downshift  command/2(engine load)
  delta gear number/1 -> current gear number/2
  gearbox speed estimator/1(Out1) -> engine torque capability/1, downshift  command/3(engine speed), upshift  command/3(engine speed)
  Constant15/1 -> Switch3/2
  [spd_dep_muxed] -> Switch3/1
  Mux/1 -> Switch3/3
  [def_gear_ratio] -> Mux/1
  [def_shifting] -> Mux/2
  Switch3/1 -> Demux/1
  Demux/1 -> "gear ratio, out"/1
  Demux/2 -> "shifting, out"/1
  Switch2/1 -> "gear number, out"/1
  Constant14/1 -> Switch2/2
  [spd_dep_gear_num] -> Switch2/1
  [def_gear_num] -> Switch2/3
  [v_req_limited] -> Speed Dependent Shifting/1
  Speed Dependent Shifting/1 -> [spd_dep_muxed]
  Speed Dependent Shifting/2 -> [spd_dep_gear_num]
  gear ratio1/1 -> [def_gear_ratio]
  shifting1/1(out_1) -> [def_shifting]

== system lib_controls/<vc> conv auto/config traction control ==
  time-average vehicle speed  req'd (m/s) : Inport
  vehicle speed at beginning of time  step (m/s) : Inport  Port=2
  total tractive force req'd (N) : Inport  Port=3
  traction control 2 axle : lib_controls/SubSystem/traction control 2 axle
  req'd force (N) : Outport
  req'd speed (m/s) : Outport  Port=2
  weight on front axle (N) : Outport  Port=3
  weight on rear axle (N) : Outport  Port=4
  front/total  traction ratio : Outport  Port=5
  wires:
  time-average vehicle speed  req'd (m/s)/1 -> traction control 2 axle/1
  vehicle speed at beginning of time  step (m/s)/1 -> traction control 2 axle/2
  total tractive force req'd (N)/1 -> traction control 2 axle/3
  traction control 2 axle/1 -> req'd force (N)/1
  traction control 2 axle/2 -> req'd speed (m/s)/1
  traction control 2 axle/3 -> weight on front axle (N)/1
  traction control 2 axle/4 -> weight on rear axle (N)/1
  traction control 2 axle/5 -> front/total  traction ratio/1

== system lib_controls/<vc> conv auto/engine control ==
  shifting : Inport
  clutch state : Inport  Port=2
  fc_spd_out_r : Inport  Port=3
  v_ave_req : Inport  Port=4
  Block NOTES : Subsystem
      mask Display: disp('Block\nNOTES')
  Constant : Constant  Value=1.1
  Constant1 : Constant  Value=vc_idle_bool
  Constant2 : Constant  Value=vc_launch_spd
  Constant3 : Constant
  Constant4 : Constant  Value=0
  Constant5 : Constant  Value=0
  Constant6 : Constant  Value=0
  Logical Operator1 : Logic
  Logical Operator2 : Logic  Operator=OR
  Logical Operator3 : Logic  Operator=OR
  Logical Operator7 : Logic
  Logical Operator8 : Logic  Inputs=3
  Memory : Memory
  Saturation : Saturate  UpperLimit=max(fc_map_spd)*fc_spd_scale  LowerLimit=vc_idle_spd*vc_idle_bool
  Switch : Switch  Threshold=eps  SaturateOnIntegerOverflow=on  InputSameDT=on
  Switch1 : Switch  Threshold=eps  SaturateOnIntegerOverflow=on  InputSameDT=on
  clutch disengaged : RelationalOperator  Operator===  InputSameDT=on
  clutch slipping or engaged : RelationalOperator  Operator=>  InputSameDT=on
  key_on : Subsystem  mask(Repeating table){t=vc_key_on(:,1), y=vc_key_on(:,2)}
      mask prompts: t "Time values:"; y "Output values:"
      mask help:
      | Repeating table.
      | Enter values of time and output for first cycle.
      mask init:
      | period = max(t);
      mask Help: Repeats cycle given in table. Time values should be monotonically increasing.
  moving next time : RelationalOperator  Operator=>  InputSameDT=on
  not moving : RelationalOperator  Operator===  InputSameDT=on
  repeated cycle:  speed required at end of NEXT step : Subsystem  mask(Forward looking repeating table){t=cyc_mph(:,1), y=cyc_mph(:,2)}
      mask prompts: t "Time values:"; y "Output values:"
      mask help:
      | Forward looking repeating table.
      | Enter values of time and output for first cycle.
      mask init:
      | period = max(t);
      mask Help: Repeats cycle given in table with a one time step forward offset. Time values should be monotonically increasing.
  engine on : Outport
  spd command  (rad/s) : Outport  Port=2
  key on : Outport  Port=3
  wires:
  key_on/1(out_1) -> key on/1, Logical Operator1/1
  Saturation/1 -> Switch1/1
  Switch1/1 -> spd command  (rad/s)/1
  Constant6/1 -> Switch1/3
  Logical Operator8/1 -> Switch/2
  fc_spd_out_r/1 -> Switch/3
  Constant2/1 -> Switch/1
  Switch/1 -> Saturation/1
  Constant5/1 -> moving next time/2
  repeated cycle:  speed required at end of NEXT step/1(out_1) -> moving next time/1
  Memory/1 -> Logical Operator7/2
  Logical Operator7/1 -> Logical Operator3/2
  shifting/1 -> Logical Operator7/1
  moving next time/1 -> Logical Operator8/3
  not moving/1 -> Logical Operator8/2
  clutch disengaged/1 -> Logical Operator8/1
  Constant4/1 -> not moving/2
  v_ave_req/1 -> not moving/1
  Constant3/1 -> clutch disengaged/2
  Logical Operator2/1 -> Logical Operator1/2
  Logical Operator3/1 -> engine on/1, Memory/1, Switch1/2
  Logical Operator1/1 -> Logical Operator3/1
  clutch slipping or engaged/1 -> Logical Operator2/1
  Constant1/1 -> Logical Operator2/2
  Constant/1 -> clutch slipping or engaged/2
  clutch state/1 -> clutch disengaged/1, clutch slipping or engaged/1

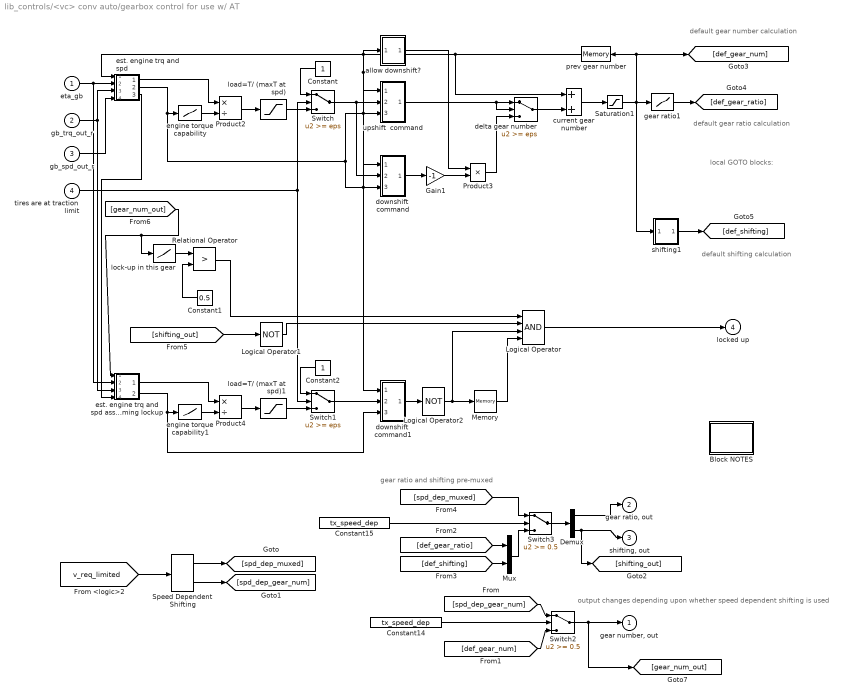
== system lib_controls/<vc> conv auto/gearbox control for use w/ AT ==
  note: default gear number
      | calculation
  note: default shifting
      | calculation
  note: default gear ratio
      | calculation
  note: local GOTO blocks:
  note: gear ratio and shifting pre-muxed
  note: output changes depending
      | upon whether speed
      | dependent shifting is used
  eta_gb : Inport
  gb_trq_out_r : Inport  Port=2
  gb_spd_out_r : Inport  Port=3
  tires are at traction limit : Inport  Port=4
  Block NOTES : Subsystem
      mask Display: disp('Block\nNOTES')
  Constant : Constant
  Constant1 : Constant  Value=0.5
  Constant14 : Constant  Value=tx_speed_dep
  Constant15 : Constant  Value=tx_speed_dep
  Constant2 : Constant
  Demux : Demux  Outputs=2
  Gain1 : Gain  Gain=-1  SaturateOnIntegerOverflow=on  OutDataTypeStr=Inherit: Same as input  ParamDataTypeStr=Inherit: Same as input
  Logical Operator : Logic  Inputs=4
  Logical Operator1 : Logic  Operator=NOT  Inputs=1
  Logical Operator2 : Logic  Operator=NOT  Inputs=1
  Memory : Memory
  Mux : Mux  Inputs=2
  Product2 : Product  Inputs=*/  SaturateOnIntegerOverflow=on  RndMeth=Zero  InputSameDT=on  OutDataTypeStr=Inherit: Same as first input
  Product3 : Product  SaturateOnIntegerOverflow=on  RndMeth=Zero  InputSameDT=on  OutDataTypeStr=Inherit: Same as first input
  Product4 : Product  Inputs=*/  SaturateOnIntegerOverflow=on  RndMeth=Zero  InputSameDT=on  OutDataTypeStr=Inherit: Same as first input
  Relational Operator : RelationalOperator  Operator=>  InputSameDT=on
  Saturation1 : Saturate  UpperLimit=gb_gears_num  LowerLimit=1
  Speed Dependent Shifting : lib_controls/SubSystem/Speed Dependent Shifting
      settings: RTWFcnNameOpts=Auto  RTWFileNameOpts=Auto
  Switch : Switch  Threshold=eps  SaturateOnIntegerOverflow=on  InputSameDT=on
  Switch1 : Switch  Threshold=eps  SaturateOnIntegerOverflow=on  InputSameDT=on
  Switch2 : Switch  Threshold=0.5  SaturateOnIntegerOverflow=on  InputSameDT=on
  Switch3 : Switch  Threshold=0.5  SaturateOnIntegerOverflow=on  InputSameDT=on
  allow downshift? : Subsystem
  current gear number : Sum  SaturateOnIntegerOverflow=on  InputSameDT=on  OutDataTypeStr=Inherit: Same as first input
  delta gear number : Switch  Threshold=eps  SaturateOnIntegerOverflow=on  InputSameDT=on
  downshift  command : Subsystem
  downshift  command1 : Subsystem
  engine torque capability : Lookup  InputValues=fc_map_spd*fc_spd_scale  Table=fc_max_trq*fc_trq_scale+eps  SaturateOnIntegerOverflow=on
  engine torque capability1 : Lookup  InputValues=fc_map_spd*fc_spd_scale  Table=fc_max_trq*fc_trq_scale+eps  SaturateOnIntegerOverflow=on
  est. engine trq and spd : Subsystem
  est. engine trq and spd assuming lockup : Subsystem
  gear ratio1 : Lookup  InputValues=[1:length(gb_ratio)]  Table=gb_ratio  SaturateOnIntegerOverflow=on
  load=T/ (maxT at spd) : Saturate  UpperLimit=1  LowerLimit=-1
  load=T/ (maxT at spd)1 : Saturate  UpperLimit=1  LowerLimit=-1
  lock-up in this gear : Lookup  InputValues=[1:length(htc_lockup)]  Table=htc_lockup  SaturateOnIntegerOverflow=on
  prev gear number : Memory  X0=gb_num_init
  shifting1 : Subsystem
  upshift  command : Subsystem
  "gear number, out" : Outport  InitialOutput=0
  "gear ratio, out" : Outport  Port=2  InitialOutput=0
  "shifting, out" : Outport  Port=3  InitialOutput=0
  locked up : Outport  Port=4  InitialOutput=0
  wires:
  est. engine trq and spd/2(est eng spd (rad/s)) -> downshift  command/3(engine speed), upshift  command/3(engine speed), engine torque capability/1
  gb_spd_out_r/1 -> est. engine trq and spd/4(gb_spd_out_r)
  Saturation1/1 -> gear ratio1/1, prev gear number/1, [def_gear_num], shifting1/1(gear number)
  Constant/1 -> Switch/1
  Product2/1 -> load=T/ (maxT at spd)/1
  allow downshift?/1(allow shift) -> Product3/1
  Product3/1 -> delta gear number/3
  engine torque capability/1 -> Product2/2
  est. engine trq and spd/1(est eng trq (Nm)) -> Product2/1
  load=T/ (maxT at spd)/1 -> Switch/3
  downshift  command/1(command) -> Gain1/1
  Logical Operator1/1 -> Logical Operator/2
  Constant1/1 -> Relational Operator/2
  lock-up in this gear/1 -> Relational Operator/1
  Relational Operator/1 -> Logical Operator/1
  Constant2/1 -> Switch1/1
  Product4/1 -> load=T/ (maxT at spd)1/1
  engine torque capability1/1 -> Product4/2
  est. engine trq and spd assuming lockup/1(est eng trq (Nm)) -> Product4/1
  eta_gb/1 -> est. engine trq and spd/2(" prev eta_gb"), est. engine trq and spd assuming lockup/2(" prev eta_gb")
  gb_trq_out_r/1 -> est. engine trq and spd/3(gb_trq_out_r), est. engine trq and spd assuming lockup/3(gb_trq_out_r)
  tires are at traction limit/1 -> Switch1/2, Switch/2
  est. engine trq and spd/3(gb_spd_in_est (rad/s)1) -> est. engine trq and spd assuming lockup/4(gb_spd_in_est)
  est. engine trq and spd assuming lockup/2(est eng spd (rad/s)) -> engine torque capability1/1, downshift  command1/3(engine speed)
  Logical Operator2/1 -> Logical Operator/3, Memory/1
  Switch/1 -> downshift  command/2(engine load), upshift  command/2(engine load)
  upshift  command/1(command) -> delta gear number/2, delta gear number/1
  Gain1/1 -> Product3/2
  Logical Operator/1 -> locked up/1
  Switch1/1 -> downshift  command1/2(engine load)
  Memory/1 -> Logical Operator/4
  load=T/ (maxT at spd)1/1 -> Switch1/3
  downshift  command1/1(command) -> Logical Operator2/1
  gear ratio1/1 -> [def_gear_ratio]
  delta gear number/1 -> current gear number/2
  current gear number/1 -> Saturation1/1
  prev gear number/1 -> current gear number/1, upshift  command/1(prev gear number), downshift  command/1(prev gear number), downshift  command1/1(prev gear number), allow downshift?/1(prev gearnum), est. engine trq and spd/1(prev gear number)
  Constant15/1 -> Switch3/2
  [spd_dep_muxed] -> Switch3/1
  Mux/1 -> Switch3/3
  [def_gear_ratio] -> Mux/1
  [def_shifting] -> Mux/2
  Switch3/1 -> Demux/1
  Constant14/1 -> Switch2/2
  [spd_dep_gear_num] -> Switch2/1
  [def_gear_num] -> Switch2/3
  [v_req_limited] -> Speed Dependent Shifting/1
  Speed Dependent Shifting/1 -> [spd_dep_muxed]
  Speed Dependent Shifting/2 -> [spd_dep_gear_num]
  Demux/2 -> "shifting, out"/1, [shifting_out]
  Switch2/1 -> "gear number, out"/1, [gear_num_out]
  shifting1/1(out_1) -> [def_shifting]
  [shifting_out] -> Logical Operator1/1
  [gear_num_out] -> lock-up in this gear/1, est. engine trq and spd assuming lockup/1(new gear number)
  Demux/1 -> "gear ratio, out"/1

== system lib_controls/<vc> conv auto Saber custom/config traction control ==
  time-average vehicle speed  req'd (m/s) : Inport
  vehicle speed at beginning of time  step (m/s) : Inport  Port=2
  total tractive force req'd (N) : Inport  Port=3
  traction control 2 axle : lib_controls/SubSystem/traction control 2 axle
      settings: RTWFcnNameOpts=Auto  RTWFileNameOpts=Auto
  req'd force (N) : Outport
  req'd speed (m/s) : Outport  Port=2
  weight on front axle (N) : Outport  Port=3
  weight on rear axle (N) : Outport  Port=4
  front/total  traction ratio : Outport  Port=5
  wires:
  time-average vehicle speed  req'd (m/s)/1 -> traction control 2 axle/1
  vehicle speed at beginning of time  step (m/s)/1 -> traction control 2 axle/2
  total tractive force req'd (N)/1 -> traction control 2 axle/3
  traction control 2 axle/1 -> req'd force (N)/1
  traction control 2 axle/2 -> req'd speed (m/s)/1
  traction control 2 axle/3 -> weight on front axle (N)/1
  traction control 2 axle/4 -> weight on rear axle (N)/1
  traction control 2 axle/5 -> front/total  traction ratio/1
